simulink model "TestMath"  (R2015b)
settings: Solver=VariableStepDiscrete  StartTime=0.0  StopTime=10.0  RelTol=1e-3
settings Model: Creator=Druzhinin_Vasily  LastModifiedBy=Druzhinin_Vasily

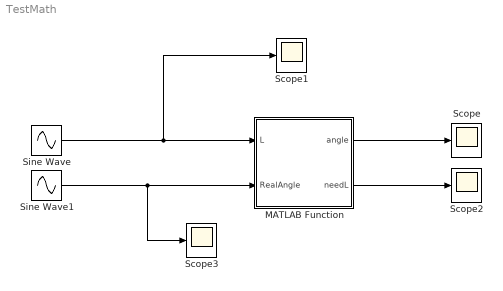
== system TestMath ==
  MATLAB Function : MATLAB Function  TreatAsAtomicUnit=on
  Scope{,1..3} (4 alike) : Scope
  Sine Wave : Sin  Amplitude=0.1  Bias=5  SampleTime=0
  Sine Wave1 : Sin  Amplitude=2.4  Bias=90  SampleTime=0
  wires:
  Sine Wave/1 -> Scope1/1, MATLAB Function/1(L)
  MATLAB Function/1(angle) -> Scope/1
  Sine Wave1/1 -> MATLAB Function/2(RealAngle), Scope3/1
  MATLAB Function/2(needL) -> Scope2/1

== matlab function TestMath/MATLAB Function ==
  data: L input; angle output; RealAngle input; needL output
function [angle,needL] = fcn(L,RealAngle)
%#codegen
a = 3;
b = 4;
angle = CalcAngles(a,b,L);
needL = Calc_L_UndoAlfa(a,b,RealAngle);
